simulink model "PlantModel"  (R2024b)
settings: Solver=VariableStepAuto  StartTime=0.0  StopTime=20  RelTol=1e-3
model workspace (MAT data in the model file):
  Drag_Constants = 1
  mass = [5.51 5.51 5.51 1 1 1]
  mass_6a = [5 5 5 1 1 1]
libraries: simulink x2
settings Model: Creator=zenyn  LastModifiedBy=zenyn
settings DebuggingCC: UnderSpecifiedDimensionMsg=warning

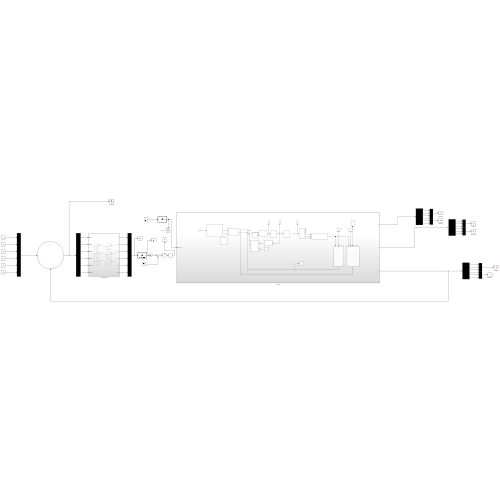
[thumbnail: Simulink's stored preview of the top-level diagram]
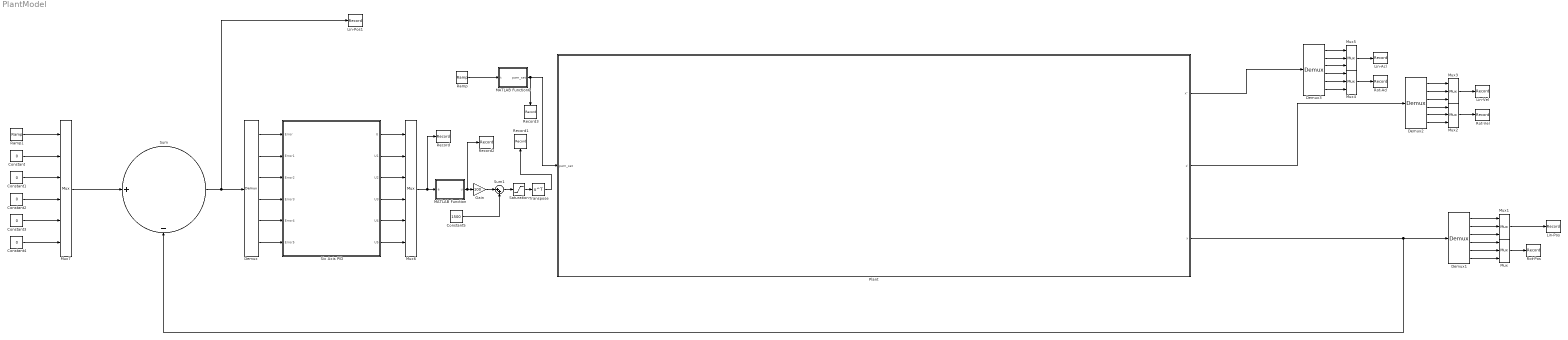
== system PlantModel ==
  Constant{,1..4} (5 alike) : Constant  Value=0
  Constant5 : Constant  Value=1500
  Demux{,1..3} (4 alike) : Demux  Outputs=6
  Gain : Gain  Gain=100
  Lin-Acl : Record  FileSettingsInternal="{\"entries\":[{\"content\":{\"excelSettings\":{\"content\":{},\"type\":\"Streamout.ExcelSettings\"}},\"type\":\"Streamout.FileSettingStorage\",\"uuid\":\"\"}],\"packageUris\":[\"http:\\/\\/schema.mathworks.com\\/mf0\\/streamout_blocks\\/R2020a\"],\"version\":\"1.0\"}"  SignalsInternal="{\"entries\":[{\"content\":{\"signals\":[{\"content\":{\"blockPath\":[],\"dimensions\":[3],\"domain\":\"\",\"hasChildren\":true,\"lineColor\":\"#d95319\",\"lineWidth\":2,\"port\":1,\"sid\":[\"\"],\"signalID\":1,\"signalName\":\"Mux5\"},\"type\":\"RecordBlkView.Signal\",\"uuid\":\"\"},{\"content\":{\"blockPath\":[],\"channel\":[1],\"dimensions\":[3],\"domain\":\"\",\"lineColor\":\"#ff6929\",\"lineWidth\":2,\"parentID\":1,\"plots\":[ 1 ],\"port\":1,\"sid\":[\"\"],\"signalID\":2,\"signalName\":\"Mux5\"},\"type\":\"RecordBlkView.Signal\",\"uuid\":\"\"},{\"content\":{\"blockPath\":[],\"channel\":[2],\"dimensions\":[3],\"domain\":\"\",\"lineColor\":\"#4dbeee\",\"lineWidth\":2,\"parentID\":1,\"plots\":[ 1 ],\"port\":1,\"sid\":[\"\"],\"signalID\":3,\"signalName\":\"Mux5\"},\"type\":\"RecordBlkView.Signal\",\"uuid\":\"\"},{\"content\":{\"blockPath\":[],\"channel\":[3],\"dimensions\":[3],\"domain\":\"\",\"lineColor\":\"#a2142f\",\"lineWidth\":2,\"parentID\":1,\"plots\":[ 1 ],\"port\":1,\"sid\":[\"\"],\"signalID\":4,\"signalName\":\"Mux5\"},\"type\":\"RecordBlkView.Signal\",\"uuid\":\"\"}]},\"type\":\"RecordBlkView.InputSignals\",\"uuid\":\"\"}],\"packageUris\":[\"http:\\/\\/schema.mathworks.com\\/mf0\\/streamout_blocks\\/R2020a\"],\"version\":\"1.0\"}"  VisualizationBindings="{\"sparklinesplugin\":{\"info\":[{\"bindingParametersList\":[],\"subplotID\":1}]}}"
  Lin-Pos : Record  FileSettingsInternal="{\"entries\":[{\"content\":{\"excelSettings\":{\"content\":{},\"type\":\"Streamout.ExcelSettings\"}},\"type\":\"Streamout.FileSettingStorage\",\"uuid\":\"\"}],\"packageUris\":[\"http:\\/\\/schema.mathworks.com\\/mf0\\/streamout_blocks\\/R2020a\"],\"version\":\"1.0\"}"  SignalsInternal="{\"entries\":[{\"content\":{\"signals\":[{\"content\":{\"blockPath\":[],\"dimensions\":[3],\"domain\":\"\",\"hasChildren\":true,\"lineColor\":\"#7e2f8e\",\"lineWidth\":2,\"port\":1,\"sid\":[\"\"],\"signalID\":1,\"signalName\":\"Mux1\"},\"type\":\"RecordBlkView.Signal\",\"uuid\":\"\"},{\"content\":{\"blockPath\":[],\"channel\":[1],\"dimensions\":[3],\"domain\":\"\",\"lineColor\":\"#64d413\",\"lineWidth\":2,\"parentID\":1,\"plots\":[ 1 ],\"port\":1,\"sid\":[\"\"],\"signalID\":2,\"signalName\":\"Mux1\"},\"type\":\"RecordBlkView.Signal\",\"uuid\":\"\"},{\"content\":{\"blockPath\":[],\"channel\":[2],\"dimensions\":[3],\"domain\":\"\",\"lineColor\":\"#139fff\",\"lineWidth\":2,\"parentID\":1,\"plots\":[ 1 ],\"port\":1,\"sid\":[\"\"],\"signalID\":3,\"signalName\":\"Mux1\"},\"type\":\"RecordBlkView.Signal\",\"uuid\":\"\"},{\"content\":{\"blockPath\":[],\"channel\":[3],\"dimensions\":[3],\"domain\":\"\",\"lineColor\":\"#ff6929\",\"lineWidth\":2,\"parentID\":1,\"plots\":[ 1 ],\"port\":1,\"sid\":[\"\"],\"signalID\":4,\"signalName\":\"Mux1\"},\"type\":\"RecordBlkView.Signal\",\"uuid\":\"\"}]},\"type\":\"RecordBlkView.InputSignals\",\"uuid\":\"\"}],\"packageUris\":[\"http:\\/\\/schema.mathworks.com\\/mf0\\/streamout_blocks\\/R2020a\"],\"version\":\"1.0\"}"  VisualizationBindings="{\"sparklinesplugin\":{\"info\":[{\"bindingParametersList\":[],\"subplotID\":1}]}}"
  Lin-Pos1 : Record  FileSettingsInternal="{\"entries\":[{\"content\":{\"excelSettings\":{\"content\":{},\"type\":\"Streamout.ExcelSettings\"}},\"type\":\"Streamout.FileSettingStorage\",\"uuid\":\"\"}],\"packageUris\":[\"http:\\/\\/schema.mathworks.com\\/mf0\\/streamout_blocks\\/R2020a\"],\"version\":\"1.0\"}"  Layout=[1 1]  SignalsInternal="{\"entries\":[{\"content\":{\"signals\":[{\"content\":{\"blockPath\":[],\"dimensions\":[1,6],\"domain\":\"\",\"hasChildren\":true,\"lineColor\":\"#4dbeee\",\"lineWidth\":2,\"port\":1,\"sid\":[\"\"],\"signalID\":1,\"signalName\":\"Sum\"},\"type\":\"RecordBlkView.Signal\",\"uuid\":\"\"},{\"content\":{\"blockPath\":[],\"channel\":[1,1],\"dimensions\":[1,6],\"domain\":\"\",\"lineColor\":\"#fe330a\",\"lineWidth\":2,\"parentID\":1,\"port\":1,\"sid\":[\"\"],\"signalID\":2,\"signalName\":\"Sum\"},\"type\":\"RecordBlkView.Signal\",\"uuid\":\"\"}]},\"type\":\"RecordBlkView.InputSignals\",\"uuid\":\"\"}],\"packageUris\":[\"http:\\/\\/schema.mathworks.com\\/mf0\\/streamout_blocks\\/R2020a\"],\"version\":\"1.0\"}"  VisualizationBindings="{\"sparklinesplugin\":{\"info\":[{\"bindingParametersList\":[],\"subplotID\":1}]}}"
  Lin-Vel : Record  FileSettingsInternal="{\"entries\":[{\"content\":{\"excelSettings\":{\"content\":{},\"type\":\"Streamout.ExcelSettings\"}},\"type\":\"Streamout.FileSettingStorage\",\"uuid\":\"\"}],\"packageUris\":[\"http:\\/\\/schema.mathworks.com\\/mf0\\/streamout_blocks\\/R2020a\"],\"version\":\"1.0\"}"  SignalsInternal="{\"entries\":[{\"content\":{\"signals\":[{\"content\":{\"blockPath\":[],\"dimensions\":[3],\"domain\":\"\",\"hasChildren\":true,\"lineColor\":\"#139fff\",\"lineWidth\":2,\"port\":1,\"sid\":[\"\"],\"signalID\":1,\"signalName\":\"Mux3\"},\"type\":\"RecordBlkView.Signal\",\"uuid\":\"\"},{\"content\":{\"blockPath\":[],\"channel\":[1],\"dimensions\":[3],\"domain\":\"\",\"lineColor\":\"#0072bd\",\"lineWidth\":2,\"parentID\":1,\"plots\":[ 1 ],\"port\":1,\"sid\":[\"\"],\"signalID\":2,\"signalName\":\"Mux3\"},\"type\":\"RecordBlkView.Signal\",\"uuid\":\"\"},{\"content\":{\"blockPath\":[],\"channel\":[2],\"dimensions\":[3],\"domain\":\"\",\"lineColor\":\"#b746ff\",\"lineWidth\":2,\"parentID\":1,\"plots\":[ 1 ],\"port\":1,\"sid\":[\"\"],\"signalID\":3,\"signalName\":\"Mux3\"},\"type\":\"RecordBlkView.Signal\",\"uuid\":\"\"},{\"content\":{\"blockPath\":[],\"channel\":[3],\"dimensions\":[3],\"domain\":\"\",\"lineColor\":\"#64d413\",\"lineWidth\":2,\"parentID\":1,\"plots\":[ 1 ],\"port\":1,\"sid\":[\"\"],\"signalID\":4,\"signalName\":\"Mux3\"},\"type\":\"RecordBlkView.Signal\",\"uuid\":\"\"}]},\"type\":\"RecordBlkView.InputSignals\",\"uuid\":\"\"}],\"packageUris\":[\"http:\\/\\/schema.mathworks.com\\/mf0\\/streamout_blocks\\/R2020a\"],\"version\":\"1.0\"}"  VisualizationBindings="{\"sparklinesplugin\":{\"info\":[{\"bindingParametersList\":[],\"subplotID\":1}]}}"
  MATLAB Function : MATLAB Function  TreatAsAtomicUnit=on
  MATLAB Function6 : MATLAB Function  TreatAsAtomicUnit=on
  Mux{,1..5} (6 alike) : Mux  Inputs=3
  Mux6 : Mux  Inputs=6
  Mux7 : Mux  Inputs=6
  Plant : Subsystem
  Ramp : simulink/Sources/Ramp  slope=1  start=0  InitialOutput=0
  Ramp1 : simulink/Sources/Ramp  slope=1  start=0  InitialOutput=0
  Record : Record  FileSettingsInternal="{\"entries\":[{\"content\":{\"excelSettings\":{\"content\":{},\"type\":\"Streamout.ExcelSettings\"}},\"type\":\"Streamout.FileSettingStorage\",\"uuid\":\"\"}],\"packageUris\":[\"http:\\/\\/schema.mathworks.com\\/mf0\\/streamout_blocks\\/R2020a\"],\"version\":\"1.0\"}"  Layout=[1 1]  SignalsInternal="{\"entries\":[{\"content\":{\"signals\":[{\"content\":{\"blockPath\":[],\"dimensions\":[6],\"domain\":\"\",\"hasChildren\":true,\"lineColor\":\"#b746ff\",\"lineWidth\":2,\"port\":1,\"sid\":[\"\"],\"signalID\":1,\"signalName\":\"Mux6\"},\"type\":\"RecordBlkView.Signal\",\"uuid\":\"\"},{\"content\":{\"blockPath\":[],\"channel\":[1],\"dimensions\":[6],\"domain\":\"\",\"lineColor\":\"#edb120\",\"lineWidth\":2,\"parentID\":1,\"port\":1,\"sid\":[\"\"],\"signalID\":2,\"signalName\":\"Mux6\"},\"type\":\"RecordBlkView.Signal\",\"uuid\":\"\"}]},\"type\":\"RecordBlkView.InputSignals\",\"uuid\":\"\"}],\"packageUris\":[\"http:\\/\\/schema.mathworks.com\\/mf0\\/streamout_blocks\\/R2020a\"],\"version\":\"1.0\"}"  VisualizationBindings="{\"sparklinesplugin\":{\"info\":[{\"bindingParametersList\":[],\"subplotID\":1}]}}"
  Record1 : Record  FileSettingsInternal="{\"entries\":[{\"content\":{\"excelSettings\":{\"content\":{},\"type\":\"Streamout.ExcelSettings\"}},\"type\":\"Streamout.FileSettingStorage\",\"uuid\":\"\"}],\"packageUris\":[\"http:\\/\\/schema.mathworks.com\\/mf0\\/streamout_blocks\\/R2020a\"],\"version\":\"1.0\"}"  Layout=[1 1]  SignalsInternal="{\"entries\":[{\"content\":{\"signals\":[{\"content\":{\"blockPath\":[],\"dimensions\":[1,8],\"domain\":\"\",\"hasChildren\":true,\"lineColor\":\"#ff13a6\",\"lineWidth\":2,\"port\":1,\"sid\":[\"\"],\"signalID\":1,\"signalName\":\"Transpose\"},\"type\":\"RecordBlkView.Signal\",\"uuid\":\"\"},{\"content\":{\"blockPath\":[],\"channel\":[1,1],\"dimensions\":[1,8],\"domain\":\"\",\"lineColor\":\"#64d413\",\"lineWidth\":2,\"parentID\":1,\"plots\":[ 1 ],\"port\":1,\"sid\":[\"\"],\"signalID\":2,\"signalName\":\"Transpose\"},\"type\":\"RecordBlkView.Signal\",\"uuid\":\"\"},{\"content\":{\"blockPath\":[],\"channel\":[1,2],\"dimensions\":[1,8],\"domain\":\"\",\"lineColor\":\"#ff13a6\",\"lineWidth\":2,\"parentID\":1,\"port\":1,\"sid\":[\"\"],\"signalID\":3,\"signalName\":\"Transpose\"},\"type\":\"RecordBlkView.Signal\",\"uuid\":\"\"},{\"content\":{\"blockPath\":[],\"channel\":[1,3],\"dimensions\":[1,8],\"domain\":\"\",\"lineColor\":\"#fe330a\",\"lineWidth\":2,\"parentID\":1,\"port\":1,\"sid\":[\"\"],\"signalID\":4,\"signalName\":\"Transpose\"},\"type\":\"RecordBlkView.Signal\",\"uuid\":\"\"},{\"content\":{\"blockPath\":[],\"channel\":[1,4],\"dimensions\":[1,8],\"domain\":\"\",\"lineColor\":\"#22b573\",\"lineWidth\":2,\"parentID\":1,\"port\":1,\"sid\":[\"\"],\"signalID\":5,\"signalName\":\"Transpose\"},\"type\":\"RecordBlkView.Signal\",\"uuid\":\"\"},{\"content\":{\"blockPath\":[],\"channel\":[1,5],\"dimensions\":[1,8],\"domain\":\"\",\"lineColor\":\"#0072bd\",\"lineWidth\":2,\"parentID\":1,\"port\":1,\"sid\":[\"\"],\"signalID\":6,\"signalName\":\"Transpose\"},\"type\":\"RecordBlkView.Signal\",\"uuid\":\"\"},{\"content\":{\"blockPath\":[],\"channel\":[1,6],\"dimensions\":[1,8],\"domain\":\"\",\"lineColor\":\"#d95319\",\"lineWidth\":2,\"parentID\":1,\"port\":1,\"sid\":[\"\"],\"signalID\":7,\"signalName\":\"Transpose\"},\"type\":\"RecordBlkView.Signal\",\"uuid\":\"\"},{\"content\":{\"blockPath\":[],\"channel\":[1,7],\"dimensions\":[1,8],\"domain\":\"\",\"lineColor\":\"#b746ff\",\"lineWidth\":2,\"parentID\":1,\"port\":1,\"sid\":[\"\"],\"signalID\":8,\"signalName\":\"Transpose\"},\"type\":\"RecordBlkView.Signal\",\"uuid\":\"\"},{\"content\":{\"blockPath\":[],\"channel\":[1,8],\"dimensions\":[1,8],\"domain\":\"\",\"lineColor\":\"#64d413\",\"lineWidth\":2,\"parentID\":1,\"port\":1,\"sid\":[\"\"],\"signalID\":9,\"signalName\":\"Transpose\"},\"type\":\"RecordBlkView.Signal\",\"uuid\":\"\"}]},\"type\":\"RecordBlkView.InputSignals\",\"uuid\":\"\"}],\"packageUris\":[\"http:\\/\\/schema.mathworks.com\\/mf0\\/streamout_blocks\\/R2020a\"],\"version\":\"1.0\"}"  VisualizationBindings="{\"sparklinesplugin\":{\"info\":[{\"bindingParametersList\":[],\"subplotID\":1}]}}"
  Record2 : Record  FileSettingsInternal="{\"entries\":[{\"content\":{\"excelSettings\":{\"content\":{},\"type\":\"Streamout.ExcelSettings\"}},\"type\":\"Streamout.FileSettingStorage\",\"uuid\":\"\"}],\"packageUris\":[\"http:\\/\\/schema.mathworks.com\\/mf0\\/streamout_blocks\\/R2020a\"],\"version\":\"1.0\"}"  Layout=[1 1]  SignalsInternal="{\"entries\":[{\"content\":{\"signals\":[{\"content\":{\"blockPath\":[],\"dimensions\":[8,1],\"domain\":\"\",\"hasChildren\":true,\"lineColor\":\"#22b573\",\"lineWidth\":2,\"port\":1,\"sid\":[\"\"],\"signalID\":1,\"signalName\":\"MATLAB Function\"},\"type\":\"RecordBlkView.Signal\",\"uuid\":\"\"},{\"content\":{\"blockPath\":[],\"channel\":[1,1],\"dimensions\":[8,1],\"domain\":\"\",\"lineColor\":\"#a2142f\",\"lineWidth\":2,\"parentID\":1,\"port\":1,\"sid\":[\"\"],\"signalID\":2,\"signalName\":\"MATLAB Function\"},\"type\":\"RecordBlkView.Signal\",\"uuid\":\"\"}]},\"type\":\"RecordBlkView.InputSignals\",\"uuid\":\"\"}],\"packageUris\":[\"http:\\/\\/schema.mathworks.com\\/mf0\\/streamout_blocks\\/R2020a\"],\"version\":\"1.0\"}"  VisualizationBindings="{\"sparklinesplugin\":{\"info\":[{\"bindingParametersList\":[],\"subplotID\":1}]}}"
  Record3 : Record  FileSettingsInternal="{\"entries\":[{\"content\":{\"excelSettings\":{\"content\":{},\"type\":\"Streamout.ExcelSettings\"}},\"type\":\"Streamout.FileSettingStorage\",\"uuid\":\"\"}],\"packageUris\":[\"http:\\/\\/schema.mathworks.com\\/mf0\\/streamout_blocks\\/R2020a\"],\"version\":\"1.0\"}"  Layout=[1 1]  SignalsInternal="{\"entries\":[{\"content\":{\"signals\":[{\"content\":{\"blockPath\":[],\"dimensions\":[1,8],\"domain\":\"\",\"hasChildren\":true,\"lineColor\":\"#d95319\",\"lineWidth\":2,\"port\":1,\"sid\":[\"\"],\"signalID\":1,\"signalName\":\"MATLAB Function6\"},\"type\":\"RecordBlkView.Signal\",\"uuid\":\"\"},{\"content\":{\"blockPath\":[],\"channel\":[1,1],\"dimensions\":[1,8],\"domain\":\"\",\"lineColor\":\"#ff6929\",\"lineWidth\":2,\"parentID\":1,\"plots\":[ 1 ],\"port\":1,\"sid\":[\"\"],\"signalID\":2,\"signalName\":\"MATLAB Function6\"},\"type\":\"RecordBlkView.Signal\",\"uuid\":\"\"},{\"content\":{\"blockPath\":[],\"channel\":[1,2],\"dimensions\":[1,8],\"domain\":\"\",\"lineColor\":\"#edb120\",\"lineWidth\":2,\"parentID\":1,\"port\":1,\"sid\":[\"\"],\"signalID\":3,\"signalName\":\"MATLAB Function6\"},\"type\":\"RecordBlkView.Signal\",\"uuid\":\"\"},{\"content\":{\"blockPath\":[],\"channel\":[1,3],\"dimensions\":[1,8],\"domain\":\"\",\"lineColor\":\"#7e2f8e\",\"lineWidth\":2,\"parentID\":1,\"port\":1,\"sid\":[\"\"],\"signalID\":4,\"signalName\":\"MATLAB Function6\"},\"type\":\"RecordBlkView.Signal\",\"uuid\":\"\"},{\"content\":{\"blockPath\":[],\"channel\":[1,4],\"dimensions\":[1,8],\"domain\":\"\",\"lineColor\":\"#77ac30\",\"lineWidth\":2,\"parentID\":1,\"port\":1,\"sid\":[\"\"],\"signalID\":5,\"signalName\":\"MATLAB Function6\"},\"type\":\"RecordBlkView.Signal\",\"uuid\":\"\"},{\"content\":{\"blockPath\":[],\"channel\":[1,5],\"dimensions\":[1,8],\"domain\":\"\",\"lineColor\":\"#4dbeee\",\"lineWidth\":2,\"parentID\":1,\"port\":1,\"sid\":[\"\"],\"signalID\":6,\"signalName\":\"MATLAB Function6\"},\"type\":\"RecordBlkView.Signal\",\"uuid\":\"\"},{\"content\":{\"blockPath\":[],\"channel\":[1,6],\"dimensions\":[1,8],\"domain\":\"\",\"lineColor\":\"#a2142f\",\"lineWidth\":2,\"parentID\":1,\"port\":1,\"sid\":[\"\"],\"signalID\":7,\"signalName\":\"MATLAB Function6\"},\"type\":\"RecordBlkView.Signal\",\"uuid\":\"\"},{\"content\":{\"blockPath\":[],\"channel\":[1,7],\"dimensions\":[1,8],\"domain\":\"\",\"lineColor\":\"#edb120\",\"lineWidth\":2,\"parentID\":1,\"port\":1,\"sid\":[\"\"],\"signalID\":8,\"signalName\":\"MATLAB Function6\"},\"type\":\"RecordBlkView.Signal\",\"uuid\":\"\"},{\"content\":{\"blockPath\":[],\"channel\":[1,8],\"dimensions\":[1,8],\"domain\":\"\",\"lineColor\":\"#7e2f8e\",\"lineWidth\":2,\"parentID\":1,\"port\":1,\"sid\":[\"\"],\"signalID\":9,\"signalName\":\"MATLAB Function6\"},\"type\":\"RecordBlkView.Signal\",\"uuid\":\"\"}]},\"type\":\"RecordBlkView.InputSignals\",\"uuid\":\"\"}],\"packageUris\":[\"http:\\/\\/schema.mathworks.com\\/mf0\\/streamout_blocks\\/R2020a\"],\"version\":\"1.0\"}"  VisualizationBindings="{\"sparklinesplugin\":{\"info\":[{\"bindingParametersList\":[],\"subplotID\":1}]}}"
  Rot-Acl : Record  FileSettingsInternal="{\"entries\":[{\"content\":{\"excelSettings\":{\"content\":{},\"type\":\"Streamout.ExcelSettings\"}},\"type\":\"Streamout.FileSettingStorage\",\"uuid\":\"\"}],\"packageUris\":[\"http:\\/\\/schema.mathworks.com\\/mf0\\/streamout_blocks\\/R2020a\"],\"version\":\"1.0\"}"  SignalsInternal="{\"entries\":[{\"content\":{\"signals\":[{\"content\":{\"blockPath\":[],\"dimensions\":[3],\"domain\":\"\",\"hasChildren\":true,\"lineColor\":\"#7e2f8e\",\"lineWidth\":2,\"port\":1,\"sid\":[\"\"],\"signalID\":1,\"signalName\":\"Mux4\"},\"type\":\"RecordBlkView.Signal\",\"uuid\":\"\"},{\"content\":{\"blockPath\":[],\"channel\":[1],\"dimensions\":[3],\"domain\":\"\",\"lineColor\":\"#64d413\",\"lineWidth\":2,\"parentID\":1,\"plots\":[ 1 ],\"port\":1,\"sid\":[\"\"],\"signalID\":2,\"signalName\":\"Mux4\"},\"type\":\"RecordBlkView.Signal\",\"uuid\":\"\"},{\"content\":{\"blockPath\":[],\"channel\":[2],\"dimensions\":[3],\"domain\":\"\",\"lineColor\":\"#ff13a6\",\"lineWidth\":2,\"parentID\":1,\"plots\":[ 1 ],\"port\":1,\"sid\":[\"\"],\"signalID\":3,\"signalName\":\"Mux4\"},\"type\":\"RecordBlkView.Signal\",\"uuid\":\"\"},{\"content\":{\"blockPath\":[],\"channel\":[3],\"dimensions\":[3],\"domain\":\"\",\"lineColor\":\"#fe330a\",\"lineWidth\":2,\"parentID\":1,\"plots\":[ 1 ],\"port\":1,\"sid\":[\"\"],\"signalID\":4,\"signalName\":\"Mux4\"},\"type\":\"RecordBlkView.Signal\",\"uuid\":\"\"}]},\"type\":\"RecordBlkView.InputSignals\",\"uuid\":\"\"}],\"packageUris\":[\"http:\\/\\/schema.mathworks.com\\/mf0\\/streamout_blocks\\/R2020a\"],\"version\":\"1.0\"}"  VisualizationBindings="{\"sparklinesplugin\":{\"info\":[{\"bindingParametersList\":[],\"subplotID\":1}]}}"
  Rot-Pos : Record  FileSettingsInternal="{\"entries\":[{\"content\":{\"excelSettings\":{\"content\":{},\"type\":\"Streamout.ExcelSettings\"}},\"type\":\"Streamout.FileSettingStorage\",\"uuid\":\"\"}],\"packageUris\":[\"http:\\/\\/schema.mathworks.com\\/mf0\\/streamout_blocks\\/R2020a\"],\"version\":\"1.0\"}"  SignalsInternal="{\"entries\":[{\"content\":{\"signals\":[{\"content\":{\"blockPath\":[],\"dimensions\":[3],\"domain\":\"\",\"hasChildren\":true,\"lineColor\":\"#4dbeee\",\"lineWidth\":2,\"port\":1,\"sid\":[\"\"],\"signalID\":1,\"signalName\":\"Mux\"},\"type\":\"RecordBlkView.Signal\",\"uuid\":\"\"},{\"content\":{\"blockPath\":[],\"channel\":[1],\"dimensions\":[3],\"domain\":\"\",\"lineColor\":\"#fe330a\",\"lineWidth\":2,\"parentID\":1,\"plots\":[ 1 ],\"port\":1,\"sid\":[\"\"],\"signalID\":2,\"signalName\":\"Mux\"},\"type\":\"RecordBlkView.Signal\",\"uuid\":\"\"},{\"content\":{\"blockPath\":[],\"channel\":[2],\"dimensions\":[3],\"domain\":\"\",\"lineColor\":\"#22b573\",\"lineWidth\":2,\"parentID\":1,\"plots\":[ 1 ],\"port\":1,\"sid\":[\"\"],\"signalID\":3,\"signalName\":\"Mux\"},\"type\":\"RecordBlkView.Signal\",\"uuid\":\"\"},{\"content\":{\"blockPath\":[],\"channel\":[3],\"dimensions\":[3],\"domain\":\"\",\"lineColor\":\"#0072bd\",\"lineWidth\":2,\"parentID\":1,\"plots\":[ 1 ],\"port\":1,\"sid\":[\"\"],\"signalID\":4,\"signalName\":\"Mux\"},\"type\":\"RecordBlkView.Signal\",\"uuid\":\"\"}]},\"type\":\"RecordBlkView.InputSignals\",\"uuid\":\"\"}],\"packageUris\":[\"http:\\/\\/schema.mathworks.com\\/mf0\\/streamout_blocks\\/R2020a\"],\"version\":\"1.0\"}"  VisualizationBindings="{\"sparklinesplugin\":{\"info\":[{\"bindingParametersList\":[],\"subplotID\":1}]}}"
  Rot-Vel : Record  FileSettingsInternal="{\"entries\":[{\"content\":{\"excelSettings\":{\"content\":{},\"type\":\"Streamout.ExcelSettings\"}},\"type\":\"Streamout.FileSettingStorage\",\"uuid\":\"\"}],\"packageUris\":[\"http:\\/\\/schema.mathworks.com\\/mf0\\/streamout_blocks\\/R2020a\"],\"version\":\"1.0\"}"  SignalsInternal="{\"entries\":[{\"content\":{\"signals\":[{\"content\":{\"blockPath\":[],\"dimensions\":[3],\"domain\":\"\",\"hasChildren\":true,\"lineColor\":\"#139fff\",\"lineWidth\":2,\"port\":1,\"sid\":[\"\"],\"signalID\":1,\"signalName\":\"Mux2\"},\"type\":\"RecordBlkView.Signal\",\"uuid\":\"\"},{\"content\":{\"blockPath\":[],\"channel\":[1],\"dimensions\":[3],\"domain\":\"\",\"lineColor\":\"#0072bd\",\"lineWidth\":2,\"parentID\":1,\"plots\":[ 1 ],\"port\":1,\"sid\":[\"\"],\"signalID\":2,\"signalName\":\"Mux2\"},\"type\":\"RecordBlkView.Signal\",\"uuid\":\"\"},{\"content\":{\"blockPath\":[],\"channel\":[2],\"dimensions\":[3],\"domain\":\"\",\"lineColor\":\"#d95319\",\"lineWidth\":2,\"parentID\":1,\"plots\":[ 1 ],\"port\":1,\"sid\":[\"\"],\"signalID\":3,\"signalName\":\"Mux2\"},\"type\":\"RecordBlkView.Signal\",\"uuid\":\"\"},{\"content\":{\"blockPath\":[],\"channel\":[3],\"dimensions\":[3],\"domain\":\"\",\"lineColor\":\"#edb120\",\"lineWidth\":2,\"parentID\":1,\"plots\":[ 1 ],\"port\":1,\"sid\":[\"\"],\"signalID\":4,\"signalName\":\"Mux2\"},\"type\":\"RecordBlkView.Signal\",\"uuid\":\"\"}]},\"type\":\"RecordBlkView.InputSignals\",\"uuid\":\"\"}],\"packageUris\":[\"http:\\/\\/schema.mathworks.com\\/mf0\\/streamout_blocks\\/R2020a\"],\"version\":\"1.0\"}"  VisualizationBindings="{\"sparklinesplugin\":{\"info\":[{\"bindingParametersList\":[],\"subplotID\":1}]}}"
  Saturation : Saturate  UpperLimit=1900  LowerLimit=1100
  Six Axis PID : Subsystem
  Sum : Sum  Inputs=|+-
  Sum1 : Sum  Inputs=|++
  Transpose : Math  Operator=transpose
  wires:
  Mux/1 -> Rot-Pos/1
  Mux1/1 -> Lin-Pos/1
  Demux1/1 -> Mux1/1
  Demux1/2 -> Mux1/2
  Demux1/3 -> Mux1/3
  Demux1/4 -> Mux/1
  Demux1/5 -> Mux/2
  Demux1/6 -> Mux/3
  Demux2/6 -> Mux2/3
  Demux2/5 -> Mux2/2
  Demux2/4 -> Mux2/1
  Demux2/3 -> Mux3/3
  Demux2/2 -> Mux3/2
  Demux2/1 -> Mux3/1
  Mux3/1 -> Lin-Vel/1
  Mux2/1 -> Rot-Vel/1
  Mux4/1 -> Rot-Acl/1
  Mux5/1 -> Lin-Acl/1
  Demux3/1 -> Mux5/1
  Demux3/2 -> Mux5/2
  Demux3/3 -> Mux5/3
  Demux3/4 -> Mux4/1
  Demux3/5 -> Mux4/2
  Demux3/6 -> Mux4/3
  Plant/1(x'') -> Demux3/1
  Plant/2(x') -> Demux2/1
  Plant/3(x) -> Demux1/1, Sum/2
  Ramp/1 -> MATLAB Function6/1(t)
  Demux/1 -> Six Axis PID/1(Error)
  Demux/2 -> Six Axis PID/2(Error1)
  Demux/3 -> Six Axis PID/3(Error2)
  Demux/4 -> Six Axis PID/4(Error3)
  Demux/5 -> Six Axis PID/5(Error4)
  Demux/6 -> Six Axis PID/6(Error5)
  Six Axis PID/1(U) -> Mux6/1
  Six Axis PID/2(U1) -> Mux6/2
  Six Axis PID/3(U2) -> Mux6/3
  Six Axis PID/4(U3) -> Mux6/4
  Six Axis PID/5(U4) -> Mux6/5
  Six Axis PID/6(U5) -> Mux6/6
  Mux6/1 -> Record/1, MATLAB Function/1(e)
  Sum/1 -> Lin-Pos1/1, Demux/1
  Mux7/1 -> Sum/1
  Ramp1/1 -> Mux7/1
  Constant/1 -> Mux7/2
  Constant1/1 -> Mux7/3
  Constant2/1 -> Mux7/4
  Constant3/1 -> Mux7/5
  Constant4/1 -> Mux7/6
  MATLAB Function/1(u) -> Record2/1, Gain/1
  Constant5/1 -> Sum1/2
  Gain/1 -> Sum1/1
  Sum1/1 -> Saturation/1
  MATLAB Function6/1(pwm_set) -> Plant/1(pwm_set), Record3/1
  Saturation/1 -> Transpose/1
  Transpose/1 -> Record1/1

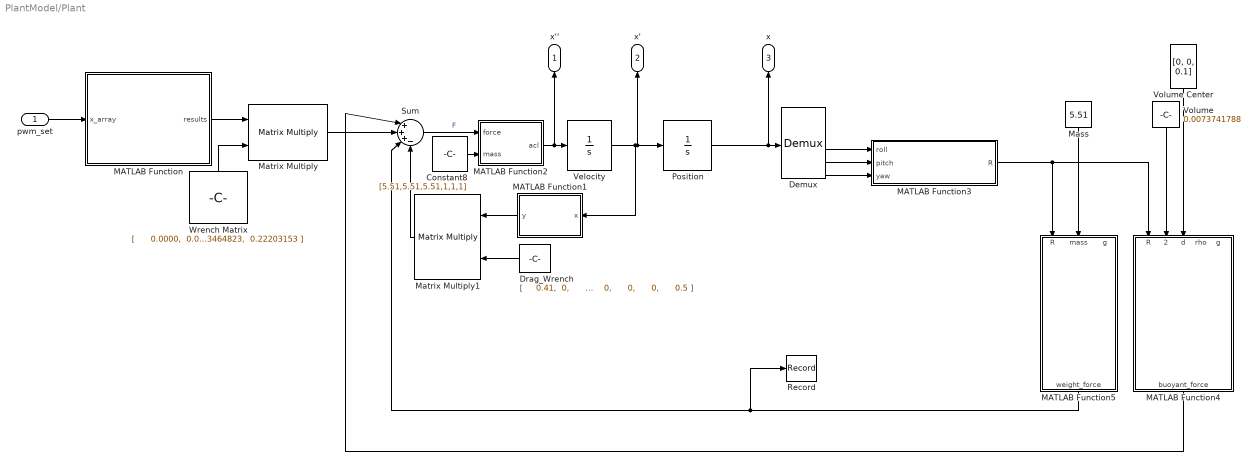
== system PlantModel/Plant ==
  pwm_set : Inport
  Constant8 : Constant  Value=[5.51,5.51,5.51,1,1,1]  VectorParams1D=off
  Demux : Demux  Outputs=6
  Drag_Wrench : Constant  Value=|  VectorParams1D=off
      | [
      |     0.41,  0,      0,      0,      0,      0;
      |     0,      0.5,   0,      0,      0,      0;
      |     0,      0,      1.25,  0,      0,      0;
      |     0,      0,      0,      0.5,   0,      0;
      |     0,      0,      0,      0,      1,    0;
      |     0,      0,      0,      0,      0,      0.5
      | ]
  MATLAB Function : MATLAB Function  TreatAsAtomicUnit=on
  MATLAB Function1 : MATLAB Function  TreatAsAtomicUnit=on
  MATLAB Function2 : MATLAB Function  TreatAsAtomicUnit=on
  MATLAB Function3 : MATLAB Function  TreatAsAtomicUnit=on
  MATLAB Function4 : MATLAB Function  TreatAsAtomicUnit=on
  MATLAB Function5 : MATLAB Function  TreatAsAtomicUnit=on
  Mass : Constant  Value=5.51
  Matrix Multiply : Product  Multiplication=Matrix(*)
  Matrix Multiply1 : Product  Multiplication=Matrix(*)
  Position : Integrator
  Record : Record  FileSettingsInternal="{\"entries\":[{\"content\":{\"excelSettings\":{\"content\":{},\"type\":\"Streamout.ExcelSettings\"}},\"type\":\"Streamout.FileSettingStorage\",\"uuid\":\"\"}],\"packageUris\":[\"http:\\/\\/schema.mathworks.com\\/mf0\\/streamout_blocks\\/R2020a\"],\"version\":\"1.0\"}"  Layout=[1 1]  SignalsInternal="{\"entries\":[{\"content\":{\"signals\":[{\"content\":{\"blockPath\":[],\"dimensions\":[1,6],\"domain\":\"\",\"hasChildren\":true,\"lineColor\":\"#ff13a6\",\"lineWidth\":2,\"port\":1,\"sid\":[\"\"],\"signalID\":1,\"signalName\":\"MATLAB Function5\"},\"type\":\"RecordBlkView.Signal\",\"uuid\":\"\"},{\"content\":{\"blockPath\":[],\"channel\":[1,1],\"dimensions\":[1,6],\"domain\":\"\",\"lineColor\":\"#b746ff\",\"lineWidth\":2,\"parentID\":1,\"plots\":[ 1 ],\"port\":1,\"sid\":[\"\"],\"signalID\":2,\"signalName\":\"MATLAB Function5\"},\"type\":\"RecordBlkView.Signal\",\"uuid\":\"\"},{\"content\":{\"blockPath\":[],\"channel\":[1,2],\"dimensions\":[1,6],\"domain\":\"\",\"lineColor\":\"#ff6929\",\"lineWidth\":2,\"parentID\":1,\"plots\":[ 1 ],\"port\":1,\"sid\":[\"\"],\"signalID\":3,\"signalName\":\"MATLAB Function5\"},\"type\":\"RecordBlkView.Signal\",\"uuid\":\"\"},{\"content\":{\"blockPath\":[],\"channel\":[1,3],\"dimensions\":[1,6],\"domain\":\"\",\"lineColor\":\"#b746ff\",\"lineWidth\":2,\"parentID\":1,\"plots\":[ 1 ],\"port\":1,\"sid\":[\"\"],\"signalID\":4,\"signalName\":\"MATLAB Function5\"},\"type\":\"RecordBlkView.Signal\",\"uuid\":\"\"},{\"content\":{\"blockPath\":[],\"channel\":[1,4],\"dimensions\":[1,6],\"domain\":\"\",\"lineColor\":\"#64d413\",\"lineWidth\":2,\"parentID\":1,\"plots\":[ 1 ],\"port\":1,\"sid\":[\"\"],\"signalID\":5,\"signalName\":\"MATLAB Function5\"},\"type\":\"RecordBlkView.Signal\",\"uuid\":\"\"},{\"content\":{\"blockPath\":[],\"channel\":[1,5],\"dimensions\":[1,6],\"domain\":\"\",\"lineColor\":\"#ff13a6\",\"lineWidth\":2,\"parentID\":1,\"plots\":[ 1 ],\"port\":1,\"sid\":[\"\"],\"signalID\":6,\"signalName\":\"MATLAB Function5\"},\"type\":\"RecordBlkView.Signal\",\"uuid\":\"\"},{\"content\":{\"blockPath\":[],\"channel\":[1,6],\"dimensions\":[1,6],\"domain\":\"\",\"lineColor\":\"#fe330a\",\"lineWidth\":2,\"parentID\":1,\"plots\":[ 1 ],\"port\":1,\"sid\":[\"\"],\"signalID\":7,\"signalName\":\"MATLAB Function5\"},\"type\":\"RecordBlkView.Signal\",\"uuid\":\"\"}]},\"type\":\"RecordBlkView.InputSignals\",\"uuid\":\"\"}],\"packageUris\":[\"http:\\/\\/schema.mathworks.com\\/mf0\\/streamout_blocks\\/R2020a\"],\"version\":\"1.0\"}"  VisualizationBindings="{\"sparklinesplugin\":{\"info\":[{\"bindingParametersList\":[],\"subplotID\":1}]}}"
  Sum : Sum  Inputs=|+++-
  Velocity : Integrator
  Volume : Constant  Value=0.0073741788
  Volume Center : Constant  Value=[0, 0, 0.1]
  Wrench Matrix : Constant  Value=|  VectorParams1D=off
      | [
      |      0.0000,  0.0000,  1.0000, -0.2035, -0.2535,  0.0000;
      |      0.0000,  0.0000,  1.0000,  0.2035, -0.2535,  0.0000;
      |      0.0000,  0.0000,  1.0000, -0.2035,  0.2545,  0.0000;
      |      0.0000,  0.0000,  1.0000,  0.2035,  0.2545,  0.0000;
      |     -0.7071, -0.7071,  0.0000, -0.03464823,  0.03464823, -0.21531401;
      |     -0.7071,  0.7071,  0.0000,  0.03464823,  0.03464823,  0.21531401;
      |     -0.7071,  0.7071,  0.0000,  0.03464823,  0.03464823, -0.22203153;
      |     -0.7071, -0.7071,  0.0000, -0.03464823,  0.03464823,  0.22203153
      | ]
  x'' : Outport
  x' : Outport  Port=2
  x : Outport  Port=3
  wires:
  Demux/4 -> MATLAB Function3/1(roll)
  Matrix Multiply/1 -> Sum/2
  Volume/1 -> MATLAB Function4/2(volume)
  Volume Center/1 -> MATLAB Function4/3(d)
  Sum/1 -> MATLAB Function2/1(force)  "F"
  Drag_Wrench/1 -> Matrix Multiply1/2
  Demux/6 -> MATLAB Function3/3(yaw)
  MATLAB Function1/1(y) -> Matrix Multiply1/1
  MATLAB Function5/1(weight_force) -> Record/1, Sum/3
  Constant8/1 -> MATLAB Function2/2(mass)
  Velocity/1 -> x'/1, Position/1, MATLAB Function1/1(x)
  MATLAB Function/1(results) -> Matrix Multiply/1
  Mass/1 -> MATLAB Function5/2(mass)
  Position/1 -> x/1, Demux/1
  Wrench Matrix/1 -> Matrix Multiply/2
  MATLAB Function3/1(R) -> MATLAB Function4/1(R), MATLAB Function5/1(R)
  MATLAB Function2/1(acl) -> x''/1, Velocity/1
  MATLAB Function4/1(buoyant_force) -> Sum/1
  Demux/5 -> MATLAB Function3/2(pitch)
  Matrix Multiply1/1 -> Sum/4
  pwm_set/1 -> MATLAB Function/1(x_array)

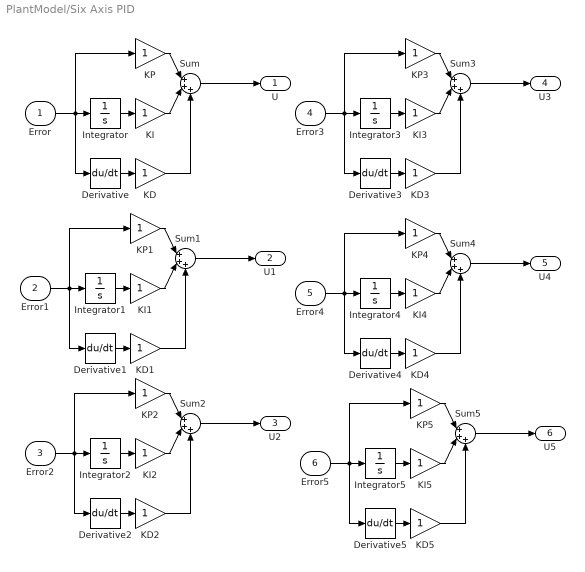
== system PlantModel/Six Axis PID ==
  Error : Inport
  Error1 : Inport  Port=2
  Error2 : Inport  Port=3
  Error3 : Inport  Port=4
  Error4 : Inport  Port=5
  Error5 : Inport  Port=6
  Derivative{,1..5} (6 alike) : Derivative
  Integrator{,1..5} (6 alike) : Integrator
  KD{,1..5} (6 alike) : Gain
  KI{,1..5} (6 alike) : Gain
  KP{,1..5} (6 alike) : Gain
  Sum{,1..5} (6 alike) : Sum  Inputs=|+++
  U : Outport
  U1 : Outport  Port=2
  U2 : Outport  Port=3
  U3 : Outport  Port=4
  U4 : Outport  Port=5
  U5 : Outport  Port=6
  wires:
  Integrator4/1 -> KI4/1
  Sum3/1 -> U3/1
  KI4/1 -> Sum4/2
  KP1/1 -> Sum1/1
  Integrator5/1 -> KI5/1
  Derivative/1 -> KD/1
  KD5/1 -> Sum5/3
  KD4/1 -> Sum4/3
  Derivative5/1 -> KD5/1
  Derivative2/1 -> KD2/1
  KI1/1 -> Sum1/2
  Integrator/1 -> KI/1
  KD/1 -> Sum/3
  KD2/1 -> Sum2/3
  Derivative3/1 -> KD3/1
  Error3/1 -> Derivative3/1, Integrator3/1, KP3/1
  KI5/1 -> Sum5/2
  KI3/1 -> Sum3/2
  KI/1 -> Sum/2
  Error5/1 -> Derivative5/1, Integrator5/1, KP5/1
  Integrator1/1 -> KI1/1
  Error/1 -> KP/1, Derivative/1, Integrator/1
  KD3/1 -> Sum3/3
  KI2/1 -> Sum2/2
  Integrator3/1 -> KI3/1
  Error2/1 -> Derivative2/1, Integrator2/1, KP2/1
  KP2/1 -> Sum2/1
  Integrator2/1 -> KI2/1
  KP4/1 -> Sum4/1
  Derivative1/1 -> KD1/1
  KD1/1 -> Sum1/3
  Error4/1 -> Derivative4/1, Integrator4/1, KP4/1
  KP3/1 -> Sum3/1
  KP/1 -> Sum/1
  KP5/1 -> Sum5/1
  Sum2/1 -> U2/1
  Sum/1 -> U/1
  Sum4/1 -> U4/1
  Sum5/1 -> U5/1
  Derivative4/1 -> KD4/1
  Sum1/1 -> U1/1
  Error1/1 -> Derivative1/1, Integrator1/1, KP1/1

== matlab function PlantModel/Plant/MATLAB Function1 ==
  data: x input; y output
function y = signed_square(x)
y = x .* abs(x);
end

== matlab function PlantModel/Plant/MATLAB Function ==
  data: x_array input; results output
function results = pwm_function(x_array)
    % Preallocate results array
    results = NaN(size(x_array)); 
    
    % First condition: 1100 <= x < 1460
    idx = (x_array >= 1100 & x_array < 1460);
    results(idx) = (-1.24422882971549e-8) * x_array(idx).^3 ...
                 + (4.02057100632393e-5) * x_array(idx).^2 ...
                 - 0.0348619861030835 * x_array(idx) ...
                 + 3.90671429105423;
    
    % Second condition: 1460 <= x <= 1540
    idx = (x_array >= 1460 & x_array <= 1540);
    results(idx) = 0;
    
    % Third condition: 1540 < x <= 1900
    idx = (x_array > 1540 & x_array <= 1900);
    results(idx) = (-1.64293565374284e-8) * x_array(idx).^3 ...
                 + (9.45962838560648e-5) * x_array(idx).^2 ...
                 - 0.170812079190679 * x_array(idx) ...
                 + 98.7232373648272;
    
    % Handle out-of-range values
    if any(isnan(results))
        error('Some values in x_array are out of the valid range [1100..1900].');
    end
end

== matlab function PlantModel/Plant/MATLAB Function2 ==
  data: force input; acl output; mass input
function acl = fcn(force, mass)
acl = force ./ mass;

end

== matlab function PlantModel/Plant/MATLAB Function3 ==
  data: roll input; R output; pitch input; yaw input
function R = rotation_matrix(roll, pitch, yaw)
    % Rotation matrix around X-axis (roll)
    Rx = [
        1,  0,           0;
        0,  cos(roll),  -sin(roll);
        0,  sin(roll),   cos(roll)
    ];

    % Rotation matrix around Y-axis (pitch)
    Ry = [
        cos(pitch),  0,  sin(pitch);
        0,           1,  0;
       -sin(pitch),  0,  cos(pitch)
    ];

    % Rotation matrix around Z-axis (yaw)
    Rz = [
        cos(yaw), -sin(yaw),  0;
        sin(yaw),  cos(yaw),  0;
        0,         0,         1
    ];

    % Combine rotations: R = Rz * Ry * Rx
    R = Rz * Ry * Rx;
end

== matlab function PlantModel/Plant/MATLAB Function4 ==
  data: R input; buoyant_force output; volume input; d input; rho input; g input
function buoyant_force = buoyant_force(R, volume, d, rho, g)
    % Set default values for fluid density and gravity if not provided
    if nargin < 6
        rho = 1000; % Default fluid density (kg/m³) for water
    end
    if nargin < 7
        g = 9.81; % Default gravitational acceleration (m/s²)
    end

    % Ensure d is a column vector
    d = d(:);

    % Buoyant force vector in world frame
    b_vector = [0; 0; rho * g * volume];

    % Rotate buoyant force to object's frame
    buoyant_force_body = R * b_vector;

    % Compute torque using cross product τ = d × F_buoyancy
    % (MATLAB cross function works for column vectors)
    torque = cross(-d, buoyant_force_body);

    % Combine force and torque into a single output vector
    buoyant_force = [buoyant_force_body; torque]';
end

== matlab function PlantModel/Plant/MATLAB Function5 ==
  data: R input; weight_force output; mass input; g input
function weight_force = weight_force(R, mass, g)
    % Set default gravitational acceleration if not provided
    if nargin < 4
        g = 9.81; % Default gravitational acceleration (m/s²)
    end

    % Gravity force vector in world frame (downward)
    g_vector = [0; 0; -mass * g];
    
    % Linear Force
    lin = R * g_vector;
    % Rotational force
    rot = [0;0;0];
    % Transform gravity force to rotated frame
    weight_force = [lin', rot'];
end

== matlab function PlantModel/MATLAB Function6 ==
  data: t input; pwm_set output
function pwm_set = fcn(t)
    rev_pulse = 1100;
    stop_pulse = 1500;
    fwd_pulse = 1900;
    
    zero_set = zeros(1, 8);
    
    stop_set = repmat(stop_pulse, 1, 8);
    
    rev_set = [repmat(stop_pulse, 1, 4), repmat(fwd_pulse, 1, 4)];
    
    fwd_set = [repmat(stop_pulse, 1, 4), repmat(rev_pulse, 1, 4)];
    
    crab_set = [repmat(stop_pulse, 1, 4), fwd_pulse, rev_pulse, rev_pulse, fwd_pulse];
    
    down_set = [repmat(rev_pulse, 1, 4), repmat(stop_pulse, 1, 4)];
    
    barrel_set = [rev_pulse, fwd_pulse, rev_pulse, fwd_pulse, repmat(stop_pulse, 1, 4)];
    
    summer_set = [rev_pulse, rev_pulse, fwd_pulse, fwd_pulse, repmat(stop_pulse, 1, 4)];
    
    spin_set = [repmat(stop_pulse, 1, 4), fwd_pulse, rev_pulse, fwd_pulse, rev_pulse];
    
    torpedo_set = [rev_pulse, fwd_pulse, rev_pulse, fwd_pulse, repmat(fwd_pulse, 1, 4)];
    
    if t < 10
        pwm_set = fwd_set;
    else
        pwm_set = rev_set;
    end
    size(pwm_set);
end

== matlab function PlantModel/MATLAB Function ==
  data: e input; u output
function u = rev_wrench(e)

wrench_matrix = [
     0.0000,  0.0000,  1.0000, -0.2035, -0.2535,  0.0000;
     0.0000,  0.0000,  1.0000,  0.2035, -0.2535,  0.0000;
     0.0000,  0.0000,  1.0000, -0.2035,  0.2545,  0.0000;
     0.0000,  0.0000,  1.0000,  0.2035,  0.2545,  0.0000;
    -0.7071, -0.7071,  0.0000, -0.03464823,  0.03464823, -0.21531401;
    -0.7071,  0.7071,  0.0000,  0.03464823,  0.03464823,  0.21531401;
    -0.7071,  0.7071,  0.0000,  0.03464823,  0.03464823, -0.22203153;
    -0.7071, -0.7071,  0.0000, -0.03464823,  0.03464823,  0.22203153];

inv_wrench = pinv(wrench_matrix);

u = inv_wrench' * -e;
end
